simulink library "vmc"  (R2021b)
settings: Solver=VariableStepAuto  StartTime=0.0  StopTime=10.0  RelTol=1e-3
undefined symbols (not defined in the file or in its folder): AVMC_ACCDeltaTqIGain_X_kph, AVMC_ACCDeltaTqIGain_Y_mps2, AVMC_ACCDeltaTqIGainP2_X_kph, AVMC_ACCDeltaTqIGainP2_Y_mps2, AVMC_ACCDeltaTqPGain_X_kph, AVMC_ACCDeltaTqPGain_Y_kph, AVMC_ACCDeltaTqPGainP2_X_kph, AVMC_ACCDeltaTqPGainP2_Y_kph, AVMC_ACCLongSteadyCtrl_X_kph, AVMC_CCAccelCMD_X_kph, AVMC_CCAccelCMD_Y_kph, AVMC_CCDeltaTqIGain_X_kph, AVMC_CCDeltaTqIGain_Y_mps2, AVMC_CCDeltaTqPGain_X_kph, AVMC_CCDeltaTqPGain_Y_kph, AVMC_CCLongSteadyCtrl_X_kph, AVMC_DISCDeltaTqIGainP2_X_kph, AVMC_DISCDeltaTqIGainP2_Y_mps2, AVMC_ESCRegenOut_X_kph, AVMC_ESCRegenOut_Y_Deg, AVMC_ESCRegenOutEnSpd_X_Deg, AVMC_LatESCRegenOut_X_kph, AVMC_LatESCRegenOut_Y_Deg, AVMC_LongAccDeadZone_X_kph, AVMC_LongAccDeadZoneP2_X_kph, AVMC_LongAccFiltTs_X_Gps, AVMC_LongAccFiltTsP2_X_Gps, AVMC_MCPresBaseTq_X_bar, AVMC_MSAAccelCMD_X_kph, AVMC_MSAAccelCMD_Y_kph, AVMC_MSADeltaTqIGain_X_kph, AVMC_MSADeltaTqIGain_Y_mps2, AVMC_MSADeltaTqPGain_X_kph, AVMC_MSADeltaTqPGain_Y_kph, AVMC_MSALongSteadyCtrl_X_kph, AVMC_MSAPedalOvrd_X_kph, AVMC_MSASpdBand_X_kph, AVMC_OPDDisSlideRate_X_Deg, AVMC_RDCDetectTime_X_kph, AVMC_RDCDetectTime_Y_pct, AVMC_RDCEnSlideRate_X_Deg, AVMC_StESCYaw_X_kph, AVMC_StESCYaw_Y_Deg, AVMC_StESCYawCom_X_kph, AVMC_StESCYawCom_Y_Gps, AVMC_TMSpdBaseTq_X_rpm, C_TASK_10MS_S, C_TASK_5MS_S, DEG2RAD, Discrete, ENUM_ADASACCSTA_ACTIVE, ENUM_ADASACCSTA_OVERRIDE, ENUM_ADASACCSTA_STANDBY, ENUM_ADASMSASTA_ACTIVE, ENUM_ADASMSASTA_ERROR, ENUM_ADASMSASTA_OFF, ENUM_ADASMSASTA_OVERSPEED, ENUM_ADASMSASTA_STANDBY, ENUM_ADASMSASTA_UNDERSPEED, ENUM_ADASMSASTA_UNLIMIT ... (+254)
libraries: hcu_lib x57, simulink x49, ctrlSharedLib x6, simulink_extras x1
(part 5 of 9)

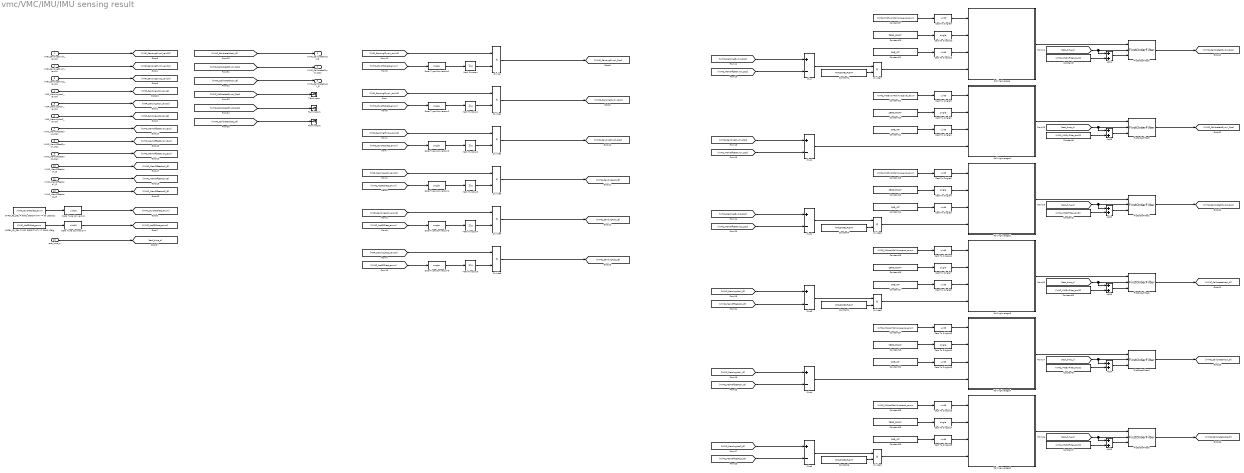
== system vmc/VMC/IMU/IMU sensing result  ==
  VINP_SensingGyroX_raw16 : Inport
  VINP_SensingGyroY_raw16 : Inport  Port=2
  VINP_SensingGyroZ_raw16 : Inport  Port=3
  VINP_SensingAccX_raw16 : Inport  Port=4
  VINP_SensingAccY_raw16 : Inport  Port=5
  VINP_SensingAccZ_raw16 : Inport  Port=6
  VVMC_MemOffsetGyroX_Dps : Inport  Port=7
  VVMC_MemOffsetGyroY_Dps : Inport  Port=8
  VVMC_MemOffsetGyroZ_Dps : Inport  Port=9
  VVMC_MemOffsetAccX_G : Inport  Port=10
  VVMC_MemOffsetAccY_G : Inport  Port=11
  VVMC_MemOffsetAccZ_G : Inport  Port=12
  task_time_s : Inport  Port=13
  ACCEL_FS_SEL = 001 SENSITIVITY = 2000 LSB/g : Constant  Value=KVMC_AccFSSlect_enum
  Add{1..5,8} (6 alike) : Sum
  Cast To Single{1,4,7,10,14,17} (6 alike) : DataTypeConversion  OutDataTypeStr=single
  Cast To Single{2..3,5..6,8..9,11..13,15..16,18} (12 alike) : DataTypeConversion  OutDataTypeStr=uint8
  Constant{1..2,4,6} (4 alike) : Constant  Value=MINUSONE_FLOAT
  Constant{10,13,16,19..20,25} (6 alike) : Constant  Value=ZERO_FLOAT
  Constant{11,14,17,21..22,26} (6 alike) : Constant  Value=ONE_INT
  Constant12 : Constant  Value=KVMC_IMUGyroYRollAveLevel_enum
  Constant15 : Constant  Value=KVMC_IMUGyroZRollAveLevel_enum
  Constant18 : Constant  Value=KVMC_IMUAccXRollAveLevel_enum
  Constant23 : Constant  Value=KVMC_IMUGxFilter_raw32
  Constant24 : Constant  Value=KVMC_IMUAccYRollAveLevel_enum
  Constant27 : Constant  Value=KVMC_IMUGyroXRollAveLevel_enum
  Constant28 : Constant  Value=KVMC_IMUAccZRollAveLevel_enum
  Constant3 : Constant  Value=KVMC_IMURxFilter_raw32
  Constant5 : Constant  Value=KVMC_IMURzFilter_raw32
  Constant7 : Constant  Value=KVMC_IMUGzFilter_raw32
  Constant8 : Constant  Value=KVMC_IMUGyFilter_raw32
  Constant9 : Constant  Value=KVMC_IMURyFilter_raw32
  Data Type Conversion : DataTypeConversion  OutDataTypeStr=uint16
  Data Type Conversion{1..6} (6 alike) : DataTypeConversion  OutDataTypeStr=single
  Data Type Conversion7 : DataTypeConversion  OutDataTypeStr=uint16
  Divide{,1..9} (10 alike) : Product  Inputs=**
  FirstOrderFilter{1..6} (6 alike) : hcu_lib/Basic_Blocks/FirstOrderFilter
  GYRO_FS_SEL = 0001 SENSITIVITY = 50 LSB/dps : Constant  Value=KVMC_GyroFSSlect_enum
  Math Function{,1..5} (6 alike) : Math  Operator=reciprocal  SaturateOnIntegerOverflow=on
  Plus{,1..5} (6 alike) : Sum  Inputs=+-
  RollingAverage : Stateflow chart  TreatAsAtomicUnit=on
  RollingAverage1 : Stateflow chart  TreatAsAtomicUnit=on
  RollingAverage2 : Stateflow chart  TreatAsAtomicUnit=on
  RollingAverage3 : Stateflow chart  TreatAsAtomicUnit=on
  RollingAverage4 : Stateflow chart  TreatAsAtomicUnit=on
  RollingAverage5 : Stateflow chart  TreatAsAtomicUnit=on
  Terminator : Terminator
  Terminator1 : Terminator
  Terminator2 : Terminator
  VVMC_CalibratedAccX_G : Outport
  VVMC_CalibratedGyroY_Dps : Outport  Port=2
  VVMC_CalibratedAccY_G : Outport  Port=3
  wires:
  Divide4/1 -> [VVMC_SensingAccY_G]  "VVMC_SensingAccY_G"
  Divide3/1 -> [VVMC_SensingAccX_G]  "VVMC_SensingAccX_G"
  Divide2/1 -> [VVMC_SensingGyroZ_Dps]  "VVMC_SensingGyroZ_Dps"
  Divide1/1 -> [VVMC_SensingGyroY_Dps]  "VVMC_SensingGyroY_Dps"
  ACCEL_FS_SEL = 001 SENSITIVITY = 2000 LSB/g/1 -> Data Type Conversion7/1
  Data Type Conversion7/1 -> [VVMC_AccFSSlect_enum]  "VVMC_AccFSSlect_enum"
  [VINP_SensingAccZ_raw16] -> Divide5/1
  [VVMC_AccFSSlect_enum] -> Data Type Conversion5/1
  [VINP_SensingAccY_raw16] -> Divide4/1
  [VINP_SensingAccX_raw16] -> Divide3/1
  [VVMC_GyroFSSlect_enum] -> Data Type Conversion3/1
  [VINP_SensingGyroZ_raw16] -> Divide2/1
  [VINP_SensingGyroY_raw16] -> Divide1/1
  [VVMC_GyroFSSlect_enum] -> Data Type Conversion2/1
  Data Type Conversion/1 -> [VVMC_GyroFSSlect_enum]  "VVMC_GyroFSSlect_enum"
  GYRO_FS_SEL = 0001 SENSITIVITY = 50 LSB/dps/1 -> Data Type Conversion/1
  [VVMC_GyroFSSlect_enum] -> Data Type Conversion1/1
  [VINP_SensingGyroX_raw16] -> Divide/1
  VVMC_MemOffsetGyroY_Dps/1 -> [VVMC_MemOffsetGyroY_Dps]
  VVMC_MemOffsetGyroX_Dps/1 -> [VVMC_MemOffsetGyroX_Dps]
  VVMC_MemOffsetAccY_G/1 -> [VVMC_MemOffsetAccY_G]
  VVMC_MemOffsetAccZ_G/1 -> [VVMC_MemOffsetAccZ_G]
  VVMC_MemOffsetGyroZ_Dps/1 -> [VVMC_MemOffsetGyroZ_Dps]
  VVMC_MemOffsetAccX_G/1 -> [VVMC_MemOffsetAccX_G]
  VINP_SensingGyroX_raw16/1 -> [VINP_SensingGyroX_raw16]
  VINP_SensingGyroY_raw16/1 -> [VINP_SensingGyroY_raw16]
  VINP_SensingGyroZ_raw16/1 -> [VINP_SensingGyroZ_raw16]
  VINP_SensingAccX_raw16/1 -> [VINP_SensingAccX_raw16]
  VINP_SensingAccY_raw16/1 -> [VINP_SensingAccY_raw16]
  VINP_SensingAccZ_raw16/1 -> [VINP_SensingAccZ_raw16]
  Divide5/1 -> [VVMC_SensingAccZ_G]  "VVMC_SensingAccZ_G"
  Divide/1 -> [VVMC_SensingGyroX_Dps]  "VVMC_SensingGyroX_Dps"
  [VVMC_SensingGyroX_Dps] -> Plus/1
  [VVMC_MemOffsetGyroX_Dps] -> Plus/2
  [VVMC_SensingGyroY_Dps] -> Plus1/1
  [VVMC_MemOffsetGyroY_Dps] -> Plus1/2
  [VVMC_SensingGyroZ_Dps] -> Plus2/1
  [VVMC_MemOffsetGyroZ_Dps] -> Plus2/2
  [VVMC_SensingAccX_G] -> Plus3/1
  [VVMC_MemOffsetAccX_G] -> Plus3/2
  [VVMC_SensingAccY_G] -> Plus4/1
  [VVMC_MemOffsetAccY_G] -> Plus4/2
  [VVMC_SensingAccZ_G] -> Plus5/1
  [VVMC_MemOffsetAccZ_G] -> Plus5/2
  FirstOrderFilter1/1 -> [VVMC_CalibratedGyroX_Dps]  "VVMC_CalibratedGyroX_Dps"
  FirstOrderFilter5/1 -> [VVMC_CalibratedGyroY_Dps]  "VVMC_CalibratedGyroY_Dps"
  FirstOrderFilter2/1 -> [VVMC_CalibratedGyroZ_Dps]  "VVMC_CalibratedGyroZ_Dps"
  FirstOrderFilter6/1 -> [VVMC_CalibratedAccX_G]  "VVMC_CalibratedAccX_G"
  FirstOrderFilter4/1 -> [VVMC_CalibratedAccY_G]  "VVMC_CalibratedAccY_G"
  FirstOrderFilter3/1 -> [VVMC_CalibratedAccZ_G]  "VVMC_CalibratedAccZ_G"
  Math Function/1 -> Divide/2
  Math Function1/1 -> Divide1/2
  Math Function2/1 -> Divide2/2
  Math Function3/1 -> Divide3/2
  Math Function4/1 -> Divide4/2
  Math Function5/1 -> Divide5/2
  Data Type Conversion1/1 -> Math Function/1
  Data Type Conversion2/1 -> Math Function1/1
  Data Type Conversion3/1 -> Math Function2/1
  [VVMC_AccFSSlect_enum] -> Data Type Conversion4/1
  Data Type Conversion4/1 -> Math Function3/1
  Data Type Conversion5/1 -> Math Function4/1
  [VVMC_AccFSSlect_enum] -> Data Type Conversion6/1
  Data Type Conversion6/1 -> Math Function5/1
  task_time_s/1 -> [task_time_s]
  [task_time_s] -> Add8/1, FirstOrderFilter6/2
  Plus3/1 -> Divide6/1
  Constant23/1 -> Add8/2
  Add8/1 -> FirstOrderFilter6/3
  Constant1/1 -> Divide6/2
  Divide6/1 -> RollingAverage3/4(VINP_INPData_raw32)
  Divide7/1 -> RollingAverage/4(VINP_INPData_raw32)
  Constant2/1 -> Divide7/2
  Add1/1 -> FirstOrderFilter1/3
  Constant3/1 -> Add1/2
  [task_time_s] -> FirstOrderFilter1/2, Add1/1
  Plus/1 -> Divide7/1
  [task_time_s] -> Add2/1, FirstOrderFilter2/2
  Constant5/1 -> Add2/2
  Add2/1 -> FirstOrderFilter2/3
  Constant4/1 -> Divide8/2
  Divide8/1 -> RollingAverage2/4(VINP_INPData_raw32)
  Plus2/1 -> Divide8/1
  Divide9/1 -> RollingAverage5/4(VINP_INPData_raw32)
  Constant6/1 -> Divide9/2
  Add3/1 -> FirstOrderFilter3/3
  Constant7/1 -> Add3/2
  [task_time_s] -> FirstOrderFilter3/2, Add3/1
  Plus5/1 -> Divide9/1
  Add4/1 -> FirstOrderFilter4/3
  Constant8/1 -> Add4/2
  [task_time_s] -> FirstOrderFilter4/2, Add4/1
  Plus4/1 -> RollingAverage4/4(VINP_INPData_raw32)
  [task_time_s] -> Add5/1, FirstOrderFilter5/2
  Constant9/1 -> Add5/2
  Add5/1 -> FirstOrderFilter5/3
  Plus1/1 -> RollingAverage1/4(VINP_INPData_raw32)
  Constant20/1 -> Cast To Single10/1
  Constant27/1 -> Cast To Single9/1
  Cast To Single12/1 -> RollingAverage/3(ONE_INT)
  Cast To Single9/1 -> RollingAverage/1(KVMC_RollAveLevel_enum)
  Cast To Single10/1 -> RollingAverage/2(ZERO_FLOAT)
  Constant21/1 -> Cast To Single12/1
  RollingAverage/1(VVMC_RollAve_raw32) -> FirstOrderFilter1/1
  Constant11/1 -> Cast To Single2/1
  Cast To Single1/1 -> RollingAverage1/2(ZERO_FLOAT)
  Cast To Single3/1 -> RollingAverage1/1(KVMC_RollAveLevel_enum)
  Cast To Single2/1 -> RollingAverage1/3(ONE_INT)
  Constant12/1 -> Cast To Single3/1
  Constant10/1 -> Cast To Single1/1
  RollingAverage1/1(VVMC_RollAve_raw32) -> FirstOrderFilter5/1
  Constant13/1 -> Cast To Single4/1
  Constant15/1 -> Cast To Single6/1
  Constant14/1 -> Cast To Single5/1
  Cast To Single6/1 -> RollingAverage2/1(KVMC_RollAveLevel_enum)
  Cast To Single4/1 -> RollingAverage2/2(ZERO_FLOAT)
  Cast To Single5/1 -> RollingAverage2/3(ONE_INT)
  RollingAverage2/1(VVMC_RollAve_raw32) -> FirstOrderFilter2/1
  Constant17/1 -> Cast To Single8/1
  Cast To Single7/1 -> RollingAverage3/2(ZERO_FLOAT)
  Cast To Single11/1 -> RollingAverage3/1(KVMC_RollAveLevel_enum)
  Cast To Single8/1 -> RollingAverage3/3(ONE_INT)
  Constant18/1 -> Cast To Single11/1
  Constant16/1 -> Cast To Single7/1
  RollingAverage3/1(VVMC_RollAve_raw32) -> FirstOrderFilter6/1
  Constant19/1 -> Cast To Single14/1
  Constant24/1 -> Cast To Single13/1
  Cast To Single15/1 -> RollingAverage4/3(ONE_INT)
  Cast To Single13/1 -> RollingAverage4/1(KVMC_RollAveLevel_enum)
  Cast To Single14/1 -> RollingAverage4/2(ZERO_FLOAT)
  Constant22/1 -> Cast To Single15/1
  RollingAverage4/1(VVMC_RollAve_raw32) -> FirstOrderFilter4/1
  Constant26/1 -> Cast To Single18/1
  Cast To Single17/1 -> RollingAverage5/2(ZERO_FLOAT)
  Cast To Single16/1 -> RollingAverage5/1(KVMC_RollAveLevel_enum)
  Cast To Single18/1 -> RollingAverage5/3(ONE_INT)
  Constant28/1 -> Cast To Single16/1
  Constant25/1 -> Cast To Single17/1
  RollingAverage5/1(VVMC_RollAve_raw32) -> FirstOrderFilter3/1
  [VVMC_CalibratedAccY_G] -> VVMC_CalibratedAccY_G/1
  [VVMC_CalibratedGyroY_Dps] -> VVMC_CalibratedGyroY_Dps/1
  [VVMC_CalibratedAccX_G] -> VVMC_CalibratedAccX_G/1
  [VVMC_CalibratedGyroX_Dps] -> Terminator/1
  [VVMC_CalibratedGyroZ_Dps] -> Terminator1/1
  [VVMC_CalibratedAccZ_G] -> Terminator2/1

== system vmc/VMC/Long Acceleration Calculation/Estimate Slope ==
  VINP_LongAccel_Gps : Inport
  VINP_VehSpeed_kph : Inport  Port=2
  task_time_s : Inport  Port=3
  VINP_GRADE_deg : Inport  Port=4
  VINP_DIDGetDynoMode_flg : Inport  Port=5
  VVMC_CalibratedAccX_G : Inport  Port=6
  AND5 : Logic  AllPortsSameDT=off  OutDataTypeStr=boolean
  Add : Sum  Inputs=+-
  Asin : Trigonometry  Operator=asin
  Constant1 : Constant  Value=KVMC_EstSlopeTs_c
  Constant14 : Constant  Value=KVMC_DIDGetDynoModeSW_flg
  Constant2 : Constant  Value=KVMC_EstSlopeTs_c
  Constant3 : Constant  Value=KVMC_EstSlopeTs_c
  Constant4 : Constant  Value=KVMC_EstSlopeSW_flg
  Constant5 : Constant  Value=KVMC_EstSlopeLongGSW_flg
  Constant6 : Constant  Value=ZERO_FLOAT
  FirstOrderFilter : hcu_lib/Basic_Blocks/FirstOrderFilter
  FirstOrderFilter1 : hcu_lib/Basic_Blocks/FirstOrderFilter
  FirstOrderFilter2 : hcu_lib/Basic_Blocks/FirstOrderFilter
  Gain : Gain  Gain=KPH2MPS
  Gain1 : Gain  Gain=1/GRAVITY_G
  Gain2 : Gain  Gain=RAD2DEG
  Switch : Switch  Criteria=u2 > Threshold
  Switch1 : Switch  Criteria=u2 > Threshold
  Switch2 : Switch  Criteria=u2 > Threshold
  derivative : hcu_lib/Basic_Blocks/derivative
  VVMC_EstSlope_Deg : Outport
  wires:
  VINP_VehSpeed_kph/1 -> FirstOrderFilter1/1
  Gain/1 -> derivative/1
  Gain1/1 -> Add/2
  Add/1 -> Asin/1  "sum"
  FirstOrderFilter/1 -> Add/1
  FirstOrderFilter1/1 -> Gain/1
  derivative/1 -> Gain1/1
  Asin/1 -> Gain2/1
  Gain2/1 -> FirstOrderFilter2/1
  FirstOrderFilter2/1 -> Switch/1  "VVMC_CalEstSlope_Deg"
  Switch1/1 -> VVMC_EstSlope_Deg/1  "VVMC_EstSlope_Deg"
  task_time_s/1 -> [task_time_s]
  [task_time_s] -> FirstOrderFilter/2
  Constant1/1 -> FirstOrderFilter/3
  [task_time_s] -> FirstOrderFilter2/2
  Constant3/1 -> FirstOrderFilter2/3
  Constant2/1 -> FirstOrderFilter1/3
  [task_time_s] -> FirstOrderFilter1/2
  Constant4/1 -> Switch/2
  VINP_GRADE_deg/1 -> Switch/3
  [task_time_s] -> derivative/2
  Constant14/1 -> AND5/2
  Switch/1 -> Switch1/3
  AND5/1 -> Switch1/2
  Constant6/1 -> Switch1/1
  VINP_DIDGetDynoMode_flg/1 -> [VINP_DIDGetDynoMode_flg]
  [VINP_DIDGetDynoMode_flg] -> AND5/1
  Switch2/1 -> FirstOrderFilter/1
  VINP_LongAccel_Gps/1 -> Switch2/3
  VVMC_CalibratedAccX_G/1 -> Switch2/1
  Constant5/1 -> Switch2/2

== system vmc/VMC/Long Acceleration Calculation/Vehicle to Meter Speed ==
  InputSpeed : Inport
  Add : Sum
  Constant1 : Constant  Value=KVMC_Veh2MetSpdAdd_kph
  Constant11 : Constant  Value=KVMC_Veh2MetSpdGain_c
  Product : Product
  OutputSpeed : Outport
  wires:
  InputSpeed/1 -> Product/1
  Product/1 -> Add/1
  Constant11/1 -> Product/2
  Add/1 -> OutputSpeed/1
  Constant1/1 -> Add/2

== system vmc/VMC/Long Acceleration Calculation/Wheel speed to long accelerate calculation ==
  VVMC_LFWhlSpeedRollAve_kph : Inport
  VVMC_RFWhlSpeedRollAve_kph : Inport  Port=2
  VVMC_LRWhlSpeedRollAve_kph : Inport  Port=3
  VVMC_RRWhlSpeedRollAve_kph : Inport  Port=4
  Add2 : Sum
  Add3 : Sum  Inputs=+-
  Constant10 : Constant  Value=KPH2MPS
  Constant11 : Constant  Value=KVMC_WSSCMDCycleTime_s
  Constant14 : Constant  Value=KVMC_GravityValue_mps2
  Constant9 : Constant  Value=KVMC_WhlSpdAvgNum_c
  Divide : Product  Inputs=*/
  Divide1 : Product  Inputs=**
  Divide2 : Product  Inputs=*/
  Divide3 : Product  Inputs=*/
  Terminator : Terminator
  Terminator1 : Terminator
  Unit Delay : UnitDelay  SampleTime=-1  HasFrameUpgradeWarning=on
  VVMC_WhlSpd2LongAcc_Gps : Outport
  wires:
  Constant11/1 -> Divide2/2
  Divide1/1 -> Divide2/1
  [VVMC_LFWhlSpeedRollAve_kph] -> Add2/1
  Constant9/1 -> Divide/2
  Divide/1 -> Add3/1, Unit Delay/1
  Divide2/1 -> Divide3/1
  [VVMC_RFWhlSpeedRollAve_kph] -> Add2/2
  Constant10/1 -> Divide1/2
  Add3/1 -> Divide1/1
  Unit Delay/1 -> Add3/2
  Add2/1 -> Divide/1
  Constant14/1 -> Divide3/2
  Divide3/1 -> VVMC_WhlSpd2LongAcc_Gps/1  "VVMC_WhlSpd2LongAcc_Gps"
  VVMC_LFWhlSpeedRollAve_kph/1 -> [VVMC_LFWhlSpeedRollAve_kph]
  VVMC_RFWhlSpeedRollAve_kph/1 -> [VVMC_RFWhlSpeedRollAve_kph]
  VVMC_LRWhlSpeedRollAve_kph/1 -> Terminator/1
  VVMC_RRWhlSpeedRollAve_kph/1 -> Terminator1/1

== system vmc/VMC/Long Acceleration Calculation/WheelSpeedRollingAverage ==
  VINP_LFRawWhlSpeed_kph : Inport
  VINP_RFRawWhlSpeed_kph : Inport  Port=2
  VINP_LRRawWhlSpeed_kph : Inport  Port=3
  VINP_RRRawWhlSpeed_kph : Inport  Port=4
  Constant : Constant  Value=ONE_INT
  Constant1 : Constant  Value=KVMC_WhlSpdRollAveLevel_enum
  Constant2 : Constant  Value=ZERO_FLOAT
  WheelSpeedRollingAverage : Stateflow chart  TreatAsAtomicUnit=on
  VVMC_LFWhlSpeedRollAve_kph : Outport
  VVMC_RFWhlSpeedRollAve_kph : Outport  Port=2
  VVMC_LRWhlSpeedRollAve_kph : Outport  Port=3
  VVMC_RRWhlSpeedRollAve_kph : Outport  Port=4
  wires:
  [VINP_LFRawWhlSpeed_kph] -> WheelSpeedRollingAverage/1(VINP_LFRawWhlSpeed_kph)
  [VINP_RRRawWhlSpeed_kph] -> WheelSpeedRollingAverage/4(VINP_RRRawWhlSpeed_kph)
  [VINP_RFRawWhlSpeed_kph] -> WheelSpeedRollingAverage/2(VINP_RFRawWhlSpeed_kph)
  WheelSpeedRollingAverage/4(VVMC_RRWhlSpeedRollAve_kph) -> [VVMC_RRWhlSpeedRollAve_kph]
  WheelSpeedRollingAverage/2(VVMC_RFWhlSpeedRollAve_kph) -> [VVMC_RFWhlSpeedRollAve_kph]
  Constant/1 -> WheelSpeedRollingAverage/5(ONE_INT)
  Constant1/1 -> WheelSpeedRollingAverage/6(KVMC_WhlSpdRollAveLevel_enum)
  [VINP_LRRawWhlSpeed_kph] -> WheelSpeedRollingAverage/3(VINP_LRRawWhlSpeed_kph)
  WheelSpeedRollingAverage/1(VVMC_LFWhlSpeedRollAve_kph) -> [VVMC_LFWhlSpeedRollAve_kph]
  Constant2/1 -> WheelSpeedRollingAverage/7(ZERO_FLOAT)
  WheelSpeedRollingAverage/3(VVMC_LRWhlSpeedRollAve_kph) -> [VVMC_LRWhlSpeedRollAve_kph]
  VINP_LRRawWhlSpeed_kph/1 -> [VINP_LRRawWhlSpeed_kph]
  VINP_RRRawWhlSpeed_kph/1 -> [VINP_RRRawWhlSpeed_kph]
  VINP_LFRawWhlSpeed_kph/1 -> [VINP_LFRawWhlSpeed_kph]
  VINP_RFRawWhlSpeed_kph/1 -> [VINP_RFRawWhlSpeed_kph]
  [VVMC_LFWhlSpeedRollAve_kph] -> VVMC_LFWhlSpeedRollAve_kph/1
  [VVMC_RFWhlSpeedRollAve_kph] -> VVMC_RFWhlSpeedRollAve_kph/1
  [VVMC_LRWhlSpeedRollAve_kph] -> VVMC_LRWhlSpeedRollAve_kph/1
  [VVMC_RRWhlSpeedRollAve_kph] -> VVMC_RRWhlSpeedRollAve_kph/1

== system vmc/VMC/LongAccel_EstSlope/Estimate Slope ==
  VINP_LongAccel_Gps : Inport
  VINP_VehSpeed_kph : Inport  Port=2
  VINP_GRADE_deg : Inport  Port=3
  Add : Sum  Inputs=+-
  Asin : Trigonometry  Operator=asin
  Constant1 : Constant  Value=KVMC_EstSlopeLongAccelTs_c
  Constant2 : Constant  Value=KVMC_EstSlopeVehSpdTs_c
  Constant3 : Constant  Value=KVMC_EstSlopeTs_c
  Constant4 : Constant  Value=KVMC_EstSlopeSW_flg
  Constant{5..8} (4 alike) : Constant  Value=C_TASK_10MS_S
  FirstOrderFilter : hcu_lib/Basic_Blocks/FirstOrderFilter
  FirstOrderFilter1 : hcu_lib/Basic_Blocks/FirstOrderFilter
  FirstOrderFilter2 : hcu_lib/Basic_Blocks/FirstOrderFilter
  Gain : Gain  Gain=KPH2MPS
  Gain1 : Gain  Gain=1/GRAVITY_G
  Gain2 : Gain  Gain=RAD2DEG
  Switch : Switch  Criteria=u2 > Threshold
  derivative : hcu_lib/Basic_Blocks/derivative
  VVMC_EstSlope_Deg : Outport
  wires:
  VINP_VehSpeed_kph/1 -> FirstOrderFilter1/1
  Gain/1 -> derivative/1
  VINP_LongAccel_Gps/1 -> FirstOrderFilter/1
  Gain1/1 -> Add/2
  Add/1 -> Asin/1  "sum"
  FirstOrderFilter/1 -> Add/1
  FirstOrderFilter1/1 -> Gain/1
  derivative/1 -> Gain1/1
  Asin/1 -> Gain2/1
  Gain2/1 -> FirstOrderFilter2/1
  FirstOrderFilter2/1 -> Switch/1
  Switch/1 -> VVMC_EstSlope_Deg/1
  Constant5/1 -> FirstOrderFilter/2
  Constant1/1 -> FirstOrderFilter/3
  Constant7/1 -> FirstOrderFilter2/2
  Constant3/1 -> FirstOrderFilter2/3
  Constant2/1 -> FirstOrderFilter1/3
  Constant6/1 -> FirstOrderFilter1/2
  Constant4/1 -> Switch/2
  VINP_GRADE_deg/1 -> Switch/3
  Constant8/1 -> derivative/2

== system vmc/VMC/LongAccel_EstSlope/VehSpdRollingAverage ==
  VINP_VehSpeed_kph : Inport
  Constant3 : Constant  Value=ONE_INT
  Constant4 : Constant  Value=KVMC_VehSpdRollAveLevel_enum
  Constant5 : Constant  Value=ZERO_FLOAT
  RollingAverage : Stateflow chart  TreatAsAtomicUnit=on
  VVMC_VehSpdRollAve_kph : Outport
  wires:
  [VVMC_VehSpdRollAve_kph] -> VVMC_VehSpdRollAve_kph/1
  VINP_VehSpeed_kph/1 -> [VINP_VehSpeed_kph]  "VINP_VehSpeed_kph"
  RollingAverage/1(VVMC_VehSpdRollAve_kph) -> [VVMC_VehSpdRollAve_kph]  "VVMC_VehSpdRollAve_kph"
  [VINP_VehSpeed_kph] -> RollingAverage/4(VINP_VehSpeed_kph)
  Constant3/1 -> RollingAverage/3(ONE_INT)
  Constant5/1 -> RollingAverage/2(ZERO_FLOAT)
  Constant4/1 -> RollingAverage/1(KVMC_VehSpdRollAveLevel_enum)

== system vmc/VMC/MSA function/Anti-Speed Limitation ==
  VINP_HoodSW_flg : Inport
  VTQD_GearActualPosn_enum : Inport  Port=2
  VINP_ZoneSpdCrlMode_enum : Inport  Port=3
  VINP_SetSpd_kph : Inport  Port=4
  AND : Logic  Inputs=3  AllPortsSameDT=off  OutDataTypeStr=boolean
  Constant1 : Constant  Value=KVMC_AntiSpdLimSW_flg
  Constant2 : Constant  Value=ENUM_GEARACTUALPOSN_D
  Constant4 : Constant  Value=3  OutDataTypeStr=uint8
  Constant5 : Constant  Value=KVMC_AntiSpdLim_kph
  Equal : RelationalOperator  Operator===  OutDataTypeStr=boolean  RndMeth=Simplest
  Switch : Switch  Criteria=u2 > Threshold
  Switch1 : Switch  Criteria=u2 > Threshold
  VVMC_AntiSpdLimEn_flg : Outport
  VVMC_MSASpdCtrlMode_enum : Outport  Port=2
  VVMC_MSASetSpd_kph : Outport  Port=3
  wires:
  [VINP_HoodSW_flg] -> AND/1
  Constant1/1 -> AND/3
  Equal/1 -> AND/2
  AND/1 -> [VVMC_AntiSpdLimEn_flg]  "VVMC_AntiSpdLimEn_flg"
  [VVMC_AntiSpdLimEn_flg] -> Switch/2
  [VINP_ZoneSpdCrlMode_enum] -> Switch/3
  [VINP_SetSpd_kph] -> Switch1/3
  Constant4/1 -> Switch/1
  [VVMC_AntiSpdLimEn_flg] -> Switch1/2
  Switch1/1 -> [VVMC_MSASetSpd_kph]  "VVMC_MSASetSpd_kph"
  Switch/1 -> [VVMC_MSASpdCtrlMode_enum]  "VVMC_MSASpdCtrlMode_enum"
  Constant2/1 -> Equal/2
  Constant5/1 -> Switch1/1
  [VTQD_GearActualPosn_enum] -> Equal/1
  VINP_HoodSW_flg/1 -> [VINP_HoodSW_flg]
  [VVMC_AntiSpdLimEn_flg] -> VVMC_AntiSpdLimEn_flg/1
  [VVMC_MSASpdCtrlMode_enum] -> VVMC_MSASpdCtrlMode_enum/1
  [VVMC_MSASetSpd_kph] -> VVMC_MSASetSpd_kph/1
  VTQD_GearActualPosn_enum/1 -> [VTQD_GearActualPosn_enum]
  VINP_ZoneSpdCrlMode_enum/1 -> [VINP_ZoneSpdCrlMode_enum]
  VINP_SetSpd_kph/1 -> [VINP_SetSpd_kph]

== system vmc/VMC/MSA function/MSAActivationHandshake ==
  VVMC_MSASpdCtrlMode_enum : Inport
  VTQD_ExternalTqAllow_flg : Inport  Port=2
  VINP_VehSpeed_kph : Inport  Port=3
  VVMC_MSASetSpd_kph : Inport  Port=4
  VINP_SWCCANCELSta_flg : Inport  Port=5
  VVMC_MSAUnLimit_flg : Inport  Port=6
  VTQD_GearActualPosn_enum : Inport  Port=7
  VINP_SWCResUpSta_flg : Inport  Port=8
  VINP_SWCSetdownSta_flg : Inport  Port=9
  VVMC_AntiSpdLimEn_flg : Inport  Port=10
  VVMC_CalMeterSpeed_kph : Inport  Port=11
  Chart : Stateflow chart  TreatAsAtomicUnit=on
  Constant : Constant  Value=KVMC_MSAActiveMetSpdHi_kph
  Constant1 : Constant  Value=KVMC_MSAActiveMetSpdLo_kph
  Constant2 : Constant  Value=KVMC_CCMSASpdWar_kph
  Constant3 : Constant  Value=ZERO_INT
  Data Type Conversion : DataTypeConversion  OutDataTypeStr=uint8
  Delay : Delay  DelayLength=1
  Detect Decrease{1..4} (4 alike) : simulink/Logic and Bit Operations/Detect Decrease  vinit=0.0  OutDataTypeStr=boolean
  Logical Operator : Logic  Operator=OR  AllPortsSameDT=off  OutDataTypeStr=boolean
  MVMC_MSASpdBand_Y_kph : Lookup_n-D  NumberOfTableDimensions=1  BreakpointsForDimension1=AVMC_MSASpdBand_X_kph  Table=MVMC_MSASpdBand_Y_kph  ExtrapMethod=Clip  InternalRulePriority=Speed  RndMeth=Simplest  InputSameDT=on
  Saturation Dynamic : simulink/Discontinuities/Saturation Dynamic  OutMin=[]  OutMax=[]  OutDataTypeStr=Inherit: Same as second input  OutDataType=fixdt(1, 16)  OutScaling=2^-10  DoSatur=off
  Switch : Switch  Criteria=u2 > Threshold
  VVMC_MSACtrlSta_enum : Outport
  VVMC_MSASpdWar_flg : Outport  Port=2
  VVMC_MSAActive_flg : Outport  Port=3
  wires:
  Chart/1(VVMC_MSACtrlSta_enum) -> [VVMC_MSACtrlSta_enum]  "VVMC_MSACtrlSta_enum"
  Chart/3(VVMC_MSAActive_flg) -> [VVMC_MSAActive_flg]  "VVMC_MSAActive_flg"
  Chart/2(VVMC_MSASpdWar_flg) -> [VVMC_MSASpdWar_flg]  "VVMC_MSASpdWar_flg"
  [VVMC_MSASpdBand_kph] -> Chart/9(VVMC_MSASpdBand_kph)
  VINP_VehSpeed_kph/1 -> [VINP_VehSpeed_kph]
  VINP_SWCCANCELSta_flg/1 -> [VINP_SWCCANCELSta_flg]
  VTQD_ExternalTqAllow_flg/1 -> [VTQD_ExternalTqAllow_flg]
  VVMC_MSASpdCtrlMode_enum/1 -> [VVMC_MSASpdCtrlMode_enum]
  [VVMC_MSAActive_flg] -> VVMC_MSAActive_flg/1
  [VVMC_MSASpdWar_flg] -> VVMC_MSASpdWar_flg/1
  [VVMC_MSACtrlSta_enum] -> VVMC_MSACtrlSta_enum/1
  [VINP_SWCCANCELSta_flg] -> Detect Decrease1/1
  Constant2/1 -> Chart/7(KVMC_CCMSASpdWar_kph)
  [VVMC_MSASetSpd_kph] -> Data Type Conversion/1
  [VINP_VehSpeed_kph] -> Chart/4(VINP_VehSpeed_kph)
  Constant/1 -> Chart/3(KVMC_MSAActiveMetSpdHi_kph)
  [VTQD_ExternalTqAllow_flg] -> Chart/2(VTQD_ExternalTqAllow_flg)
  [VVMC_MSASpdCtrlMode_enum] -> Chart/1(VVMC_MSASpdCtrlMode_enum)
  [VVMC_MSAUnLimit_flg] -> Delay/1
  Delay/1 -> Chart/10(VVMC_MSAUnLimit_flg)
  VVMC_MSAUnLimit_flg/1 -> [VVMC_MSAUnLimit_flg]
  VTQD_GearActualPosn_enum/1 -> [VTQD_GearActualPosn_enum]
  [VTQD_GearActualPosn_enum] -> Chart/11(VTQD_GearActualPosn_enum)
  Saturation Dynamic/1 -> [VVMC_MSASpdBand_kph]  "VVMC_MSASpdBand_kph"
  MVMC_MSASpdBand_Y_kph/1 -> Saturation Dynamic/2
  Constant3/1 -> Saturation Dynamic/3
  VINP_SWCSetdownSta_flg/1 -> [VINP_SWCSetdownSta_flg]
  VINP_SWCResUpSta_flg/1 -> [VINP_SWCResUpSta_flg]
  Detect Decrease2/1 -> Chart/12(VINP_SWCResUpSta_flg)
  Detect Decrease3/1 -> Chart/13(VINP_SWCSetdownSta_flg)
  [VINP_SWCResUpSta_flg] -> Detect Decrease2/1
  [VINP_SWCSetdownSta_flg] -> Detect Decrease3/1
  VVMC_AntiSpdLimEn_flg/1 -> [VVMC_AntiSpdLimEn_flg]
  Switch/1 -> Chart/5(VVMC_MSAActiveMetSpdLo_kph)
  [VVMC_MSASetSpd_kph] -> Switch/1
  [VVMC_AntiSpdLimEn_flg] -> Switch/2
  Constant1/1 -> Switch/3
  Data Type Conversion/1 -> Chart/6(VVMC_MSASetSpd_kph)
  [VVMC_MSASetSpd_kph] -> MVMC_MSASpdBand_Y_kph/1
  [VVMC_MSASetSpd_kph] -> Saturation Dynamic/1
  VVMC_MSASetSpd_kph/1 -> [VVMC_MSASetSpd_kph]
  [VVMC_AntiSpdLimEn_flg] -> Chart/14(VVMC_AntiSpdLimEn_flg)
  Logical Operator/1 -> Chart/8(VVMC_DetectSWCCANCEL_flg)  "VVMC_DetectSWCCANCEL_flg"
  [VVMC_AntiSpdLimEn_flg] -> Detect Decrease4/1
  Detect Decrease1/1 -> Logical Operator/1
  Detect Decrease4/1 -> Logical Operator/2
  VVMC_CalMeterSpeed_kph/1 -> [VVMC_CalMeterSpeed_kph]
  [VVMC_CalMeterSpeed_kph] -> Chart/15(VVMC_CalMeterSpeed_kph)

== system vmc/VMC/MSA function/MSADemandTorqueCalculation ==
  VVMC_MSASetSpd_kph : Inport
  VVMC_MSAActive_flg : Inport  Port=2
  VTQD_DriverWhlTqDem_Nm : Inport  Port=3
  VVMC_LongAcc_Gps : Inport  Port=4
  VVMC_MSAUnLimit_flg : Inport  Port=5
  VVMC_CalMeterSpeed_kph : Inport  Port=6
  " MSA Acceleration Determination" : Lookup_n-D  BreakpointsForDimension1=AVMC_MSAAccelCMD_Y_kph  BreakpointsForDimension2=AVMC_MSAAccelCMD_X_kph  BreakpointsForDimension3=[5, 7]  Table=MVMC_MSAAccelCMD_Z_mps2  ExtrapMethod=Clip  InternalRulePriority=Speed  RndMeth=Simplest  InputSameDT=on
      settings: InputPortMap=u0,u1
  Abs : Abs
  Add : Sum  Inputs=+-
  Add{1..2,5..6} (4 alike) : Sum
  Add3 : Sum  Inputs=+-
  Add4 : Sum  Inputs=+-
  Constant : Constant  Value=KVMC_MSAInitTqDEM_Nm
  Constant1 : Constant  Value=KVMC_MSAAccelCMDUpLim_mps2
  Constant10 : Constant  Value=KVMC_GravityValue_mps2
  Constant11 : Constant  Value=KVMC_MSADevLowLim_mps2
  Constant12 : Constant  Value=ZERO_INT
  Constant13 : Constant  Value=KVMC_MSAPGainTqSW_flg
  Constant14 : Constant  Value=KVMC_MSAPGainTqSW_flg
  Constant15 : Constant  Value=ZERO_INT
  Constant16 : Constant  Value=ZERO_INT
  Constant19 : Constant  Value=KVMC_MSADevUpLim_mps2
  Constant2 : Constant  Value=KVMC_MSAAccelCMDLowLim_mps2
  Constant3 : Constant  Value=KVMC_MSATqUpLim_Nm  OutDataTypeStr=single
  Constant4 : Constant  Value=KVMC_MSATqLowLim_Nm  OutDataTypeStr=single
  Constant5 : Constant  Value=KVMC_MSAPedalOvrdSetSpd_kph
  Constant6 : Constant  Value=KVMC_MSAIGainOffDevSpd_kph
  Constant7 : Constant  Value=KVMC_MSASpdDevUpLim_kph
  Constant8 : Constant  Value=KVMC_MSASpdDevLowLim_kph
  Detect Increase : simulink/Logic and Bit Operations/Detect Increase  vinit=0.0  OutDataTypeStr=boolean
  MVMC_MSADeltaTqIGain_Z_Nm : Lookup_n-D  BreakpointsForDimension1=AVMC_MSADeltaTqIGain_Y_mps2  BreakpointsForDimension2=AVMC_MSADeltaTqIGain_X_kph  Table=MVMC_MSADeltaTqIGain_Z_Nm  ExtrapMethod=Clip  InternalRulePriority=Speed  RndMeth=Simplest  InputSameDT=on
      settings: InputPortMap=u0,u1
  MVMC_MSADeltaTqPGain_Z_Nm : Lookup_n-D  BreakpointsForDimension1=AVMC_MSADeltaTqPGain_Y_kph  BreakpointsForDimension2=AVMC_MSADeltaTqPGain_X_kph  BreakpointsForDimension3=[5, 7]  Table=MVMC_MSADeltaTqPGain_Z_Nm  ExtrapMethod=Clip  InternalRulePriority=Speed  RndMeth=Simplest  InputSameDT=on
      settings: InputPortMap=u0,u1
  Product : Product
  Relational Operator : RelationalOperator  Operator=<  OutDataTypeStr=boolean  RndMeth=Simplest
  Saturation Dynamic{,1..2,4} (4 alike) : simulink/Discontinuities/Saturation Dynamic  OutMin=[]  OutMax=[]  OutDataTypeStr=Inherit: Same as second input  OutDataType=fixdt(1, 16)  OutScaling=2^-10  DoSatur=off
  Switch : Switch  Criteria=u2 ~= 0
  Switch1 : Switch  Criteria=u2 ~= 0
  Switch{2..5,7} (5 alike) : Switch  Criteria=u2 > Threshold
  Unit Delay : UnitDelay  SampleTime=-1  HasFrameUpgradeWarning=on
  VVMC_MSAWhlTqCal_Nm : Outport
  wires:
  Switch3/1 -> Add5/1  "VVMC_MSADeltaTqIGain_Nm"
  Add5/1 -> [VVMC_MSADeltaTq_Nm]  "VVMC_MSADeltaTq_Nm"
  Saturation Dynamic4/1 -> [VVMC_MSAActSpdDev_kph], MVMC_MSADeltaTqPGain_Z_Nm/1  "VVMC_MSAActSpdDev_kph"
  Constant8/1 -> Saturation Dynamic4/3
  Constant7/1 -> Saturation Dynamic4/1
  Add4/1 -> Saturation Dynamic4/2
  Add6/1 -> [VVMC_MSAWhlTqCal_Nm]  "VVMC_MSAWhlTqCal_Nm"
  Constant4/1 -> Saturation Dynamic/3
  Switch1/1 -> Saturation Dynamic/2
  Saturation Dynamic2/1 -> [VVMC_MSAAccelCMD_mps2]  "VVMC_MSAAccelCMD_mps2"
  " MSA Acceleration Determination"/1 -> Saturation Dynamic2/2
  Constant1/1 -> Saturation Dynamic2/1
  Constant2/1 -> Saturation Dynamic2/3
  Add3/1 -> Saturation Dynamic1/2
  [VVMC_LongAcc_Gps] -> Product/1
  Constant10/1 -> Product/2
  Constant19/1 -> Saturation Dynamic1/1
  Saturation Dynamic1/1 -> MVMC_MSADeltaTqIGain_Z_Nm/1  "VVMC_ActMSAAccDev_mps2"
  Product/1 -> Add3/2
  Constant11/1 -> Saturation Dynamic1/3
  [VVMC_MSAAccelCMD_mps2] -> Add3/1
  VVMC_LongAcc_Gps/1 -> [VVMC_LongAcc_Gps]
  VTQD_DriverWhlTqDem_Nm/1 -> [VTQD_DriverWhlTqDem_Nm]
  VVMC_MSAActive_flg/1 -> [VVMC_MSAActive_flg]
  VVMC_MSASetSpd_kph/1 -> [VVMC_MSASetSpd_kph]
  [VVMC_MSAWhlTqCal_Nm] -> VVMC_MSAWhlTqCal_Nm/1
  [VVMC_MSADeltaTq_Nm] -> Add2/2
  [VVMC_MSADeltaTq_Nm] -> Add1/2
  Switch/1 -> Switch1/1
  Add2/1 -> Switch/3
  Unit Delay/1 -> [VVMC_MSAWhlTqCalDelay_Nm]  "VVMC_MSAWhlTqCalDelay_Nm"
  Detect Increase/1 -> Switch/2
  [VVMC_MSAActive_flg] -> Switch1/2
  [VVMC_MSAActive_flg] -> Detect Increase/1
  Add1/1 -> Switch/1
  [VVMC_MSAWhlTqCalDelay_Nm] -> Add2/1
  [VTQD_DriverWhlTqDem_Nm] -> Add1/1
  Constant/1 -> Switch1/3
  Add/1 -> " MSA Acceleration Determination"/1
  VVMC_MSAUnLimit_flg/1 -> [VVMC_MSAUnLimit_flg]
  [VVMC_MSAUnLimit_flg] -> Switch2/2
  Constant5/1 -> Switch2/1
  Switch2/1 -> [VVMC_ActMSASetSpd_kph]  "VVMC_ActMSASetSpd_kph"
  [VVMC_ActMSASetSpd_kph] -> Add/1
  [VVMC_ActMSASetSpd_kph] -> Add4/1
  [VVMC_CalMeterSpeed_kph] -> Add/2
  [VVMC_CalMeterSpeed_kph] -> Add4/2
  VVMC_CalMeterSpeed_kph/1 -> [VVMC_CalMeterSpeed_kph]
  [VVMC_ActMSASetSpd_kph] -> " MSA Acceleration Determination"/2
  [VVMC_ActMSASetSpd_kph] -> MVMC_MSADeltaTqIGain_Z_Nm/2
  [VVMC_ActMSASetSpd_kph] -> MVMC_MSADeltaTqPGain_Z_Nm/2
  Constant3/1 -> Switch7/3
  [VVMC_MSAActive_flg] -> Switch7/2
  Switch7/1 -> Saturation Dynamic/1  "VVMC_MSATqUpLim_Nm"
  [VTQD_DriverWhlTqDem_Nm] -> Switch7/1
  [VVMC_MSASetSpd_kph] -> Switch2/3
  Switch4/1 -> Add6/1
  Constant14/1 -> Switch4/2
  [VVMC_MSADeltaTqPGain_Nm] -> Switch4/1
  Constant15/1 -> Switch4/3
  Saturation Dynamic/1 -> Unit Delay/1, Add6/2
  MVMC_MSADeltaTqPGain_Z_Nm/1 -> [VVMC_MSADeltaTqPGain_Nm]  "VVMC_MSADeltaTqPGain_Nm"
  [VVMC_MSADeltaTqPGain_Nm] -> Switch5/3
  Switch5/1 -> Add5/2
  Constant13/1 -> Switch5/2
  Constant16/1 -> Switch5/1
  Relational Operator/1 -> Switch3/2
  Abs/1 -> Relational Operator/1
  Constant6/1 -> Relational Operator/2
  [VVMC_MSAActSpdDev_kph] -> Abs/1
  Constant12/1 -> Switch3/1
  MVMC_MSADeltaTqIGain_Z_Nm/1 -> Switch3/3

== system vmc/VMC/MSA function/MSATorqueSourceDetermination ==
  VVMC_MSAWhlTqCal_Nm : Inport
  VTQD_DriverWhlTqDem_Nm : Inport  Port=2
  VVMC_MSACtrlSta_enum : Inport  Port=3
  VVMC_MSAActive_flg : Inport  Port=4
  VINP_VehSpeed_kph : Inport  Port=5
  VVMC_MSASetSpd_kph : Inport  Port=6
  task_time_s : Inport  Port=7
  VDHP_ActAPSPosn_pct : Inport  Port=8
  VVMC_AntiSpdLimEn_flg : Inport  Port=9
  AND : Logic  Inputs=3  AllPortsSameDT=off  OutDataTypeStr=boolean
  AND{2..6} (5 alike) : Logic  AllPortsSameDT=off  OutDataTypeStr=boolean
  Add1 : Sum  Inputs=+-
  Constant1 : Constant  Value=KVMC_MSAUnLimitDetTime_s
  Constant10 : Constant  Value=KVMC_MSAUnLimitResetTime_s
  Constant14 : Constant  Value=KVMC_MSAPedOvrdTqConTq_Nm
  Constant15 : Constant  Value=ENUM_ADASMSASTA_ACTIVE
  Constant3 : Constant  Value=ENUM_ADASMSASTA_ACTIVE
  Delay3 : Delay  DelayLength=1
  Detect Decrease : simulink/Logic and Bit Operations/Detect Decrease  vinit=0.0  OutDataTypeStr=boolean
  Detect Increase1 : simulink/Logic and Bit Operations/Detect Increase  vinit=0.0  OutDataTypeStr=boolean
  Equal1 : RelationalOperator  Operator===  OutDataTypeStr=boolean  RndMeth=Simplest
  Equal2 : RelationalOperator  Operator===  OutDataTypeStr=boolean  RndMeth=Simplest
  MVMC_MSAPedalOvrd_Y_pct : Lookup_n-D  NumberOfTableDimensions=1  BreakpointsForDimension1=AVMC_MSAPedalOvrd_X_kph  Table=MVMC_MSAPedalOvrd_Y_pct  ExtrapMethod=Clip  InternalRulePriority=Speed  RndMeth=Simplest  InputSameDT=on
  NOT{,2..5} (5 alike) : Logic  Operator=NOT  AllPortsSameDT=off  OutDataTypeStr=boolean
  OR : Logic  Operator=OR  Inputs=3  AllPortsSameDT=off  OutDataTypeStr=boolean
  OR3 : Logic  Operator=OR  AllPortsSameDT=off  OutDataTypeStr=boolean
  Relational Operator : RelationalOperator  OutDataTypeStr=boolean  RndMeth=Simplest
  Relational Operator1 : RelationalOperator  Operator=>  OutDataTypeStr=boolean  RndMeth=Simplest
  Relational Operator2 : RelationalOperator  OutDataTypeStr=boolean  RndMeth=Simplest
  Relational Operator3 : RelationalOperator  Operator=<=  OutDataTypeStr=boolean  RndMeth=Simplest
  Relational Operator4 : RelationalOperator  OutDataTypeStr=boolean  RndMeth=Simplest
  Relational Operator5 : RelationalOperator  Operator=<=  OutDataTypeStr=boolean  RndMeth=Simplest
  SR_Latch1 : hcu_lib/Basic_Blocks/SR_Latch
  SR_Latch2 : hcu_lib/Basic_Blocks/SR_Latch
  Switch : Switch  Criteria=u2 ~= 0
  Timer : hcu_lib/Basic_Blocks/Timer
  Timer1 : hcu_lib/Basic_Blocks/Timer
  VVMC_MSAWhlTqReq_Nm : Outport
  VVMC_MSAUnLimit_flg : Outport  Port=2
  wires:
  [VVMC_MSAWhlTqCal_Nm] -> Relational Operator/1
  [VTQD_DriverWhlTqDem_Nm] -> Relational Operator/2
  [VTQD_DriverWhlTqDem_Nm] -> Switch/1
  [VVMC_MSAWhlTqCal_Nm] -> Switch/3
  Switch/1 -> [VVMC_MSAWhlTqReq_Nm]  "VVMC_MSAWhlTqReq_Nm"
  [VVMC_MSAWhlTqReq_Nm] -> VVMC_MSAWhlTqReq_Nm/1
  VVMC_MSAWhlTqCal_Nm/1 -> [VVMC_MSAWhlTqCal_Nm]
  VTQD_DriverWhlTqDem_Nm/1 -> [VTQD_DriverWhlTqDem_Nm]
  Constant1/1 -> Relational Operator2/2, Timer/4
  VVMC_MSACtrlSta_enum/1 -> [VVMC_MSACtrlSta_enum]
  Timer/1 -> Relational Operator2/1  "VVMC_MSAUnLimitDetTime_s"
  Relational Operator2/1 -> [VVMC_MSAUnLimitDetFinish_flg]  "VVMC_MSAUnLimitDetFinish_flg"
  NOT/1 -> Timer/2
  [task_time_s] -> Timer/3
  SR_Latch1/1 -> [VVMC_MSAUnLimit_flg]  "VVMC_MSAUnLimit_flg"
  [VINP_VehSpeed_kph] -> Relational Operator3/1
  NOT2/1 -> OR/1
  [VVMC_MSAActive_flg] -> NOT2/1
  OR/1 -> SR_Latch1/2  "VVMC_MASUnLimitDis_flg"
  OR3/1 -> Switch/2  "VVMC_MSAChangeToPedal_flg"
  [VVMC_ActMSAUnLimit_flg] -> OR3/2
  VVMC_MSAActive_flg/1 -> [VVMC_MSAActive_flg]
  VINP_VehSpeed_kph/1 -> [VINP_VehSpeed_kph]
  VVMC_MSASetSpd_kph/1 -> [VVMC_MSASetSpd_kph]
  task_time_s/1 -> [task_time_s]
  [VVMC_MSAUnLimit_flg] -> VVMC_MSAUnLimit_flg/1
  AND2/1 -> OR/2
  Relational Operator3/1 -> AND2/1
  [VVMC_MSAUnLimit_flg] -> Delay3/1
  Delay3/1 -> Timer1/1, NOT3/1
  NOT3/1 -> Timer1/2
  [task_time_s] -> Timer1/3
  Constant10/1 -> Relational Operator4/2, Timer1/4
  Timer1/1 -> Relational Operator4/1  "VVMC_MSAUnLimitResetTime_s"
  Relational Operator4/1 -> [VVMC_MSAUnLimitReset_flg]  "VVMC_MSAUnLimitReset_flg"
  [VVMC_MSAUnLimitReset_flg] -> AND2/2
  VDHP_ActAPSPosn_pct/1 -> [VDHP_ActAPSPosn_pct]
  MVMC_MSAPedalOvrd_Y_pct/1 -> Relational Operator1/2  "VVMC_MSAPedalOvrd_pct"
  [VDHP_ActAPSPosn_pct] -> Relational Operator1/1
  [VVMC_MSAUnLimitDetFinish_flg] -> SR_Latch1/1
  [VTQD_DriverWhlTqDem_Nm] -> Add1/1
  [VVMC_MSAWhlTqCal_Nm] -> Add1/2
  [VVMC_MSAUnLimit_flg] -> AND3/2
  Relational Operator5/1 -> AND3/1
  Constant14/1 -> Relational Operator5/2
  Add1/1 -> Relational Operator5/1
  Relational Operator/1 -> AND4/2
  NOT4/1 -> AND4/1
  [VVMC_MSAUnLimit_flg] -> NOT4/1
  AND4/1 -> OR3/1
  Relational Operator1/1 -> AND5/1, Detect Increase1/1, Detect Decrease/1
  SR_Latch2/1 -> AND5/2  "VVMC_MSAInstPedOvrd_flg"
  Detect Decrease/1 -> SR_Latch2/2
  Constant15/1 -> Equal1/2
  [VVMC_MSACtrlSta_enum] -> Equal1/1
  AND6/1 -> SR_Latch2/1
  Detect Increase1/1 -> AND6/1
  Equal1/1 -> AND6/2
  AND5/1 -> [VVMC_MSAPedalOvrd_flg]  "VVMC_MSAPedalOvrd_flg"
  [VVMC_MSASetSpd_kph] -> MVMC_MSAPedalOvrd_Y_pct/1
  [VVMC_MSASetSpd_kph] -> Relational Operator3/2
  VVMC_AntiSpdLimEn_flg/1 -> [VVMC_AntiSpdLimEn_flg]
  AND3/1 -> [VVMC_ActMSAUnLimit_flg]  "VVMC_ActMSAUnLimit_flg"
  [VVMC_AntiSpdLimEn_flg] -> NOT5/1
  Constant3/1 -> Equal2/2
  [VVMC_MSAPedalOvrd_flg] -> AND/1
  AND/1 -> NOT/1, Timer/1  "VVMC_UnLimitTimerEn_flg"
  Equal2/1 -> AND/3
  NOT5/1 -> AND/2
  [VVMC_MSACtrlSta_enum] -> Equal2/1
  [VVMC_AntiSpdLimEn_flg] -> OR/3

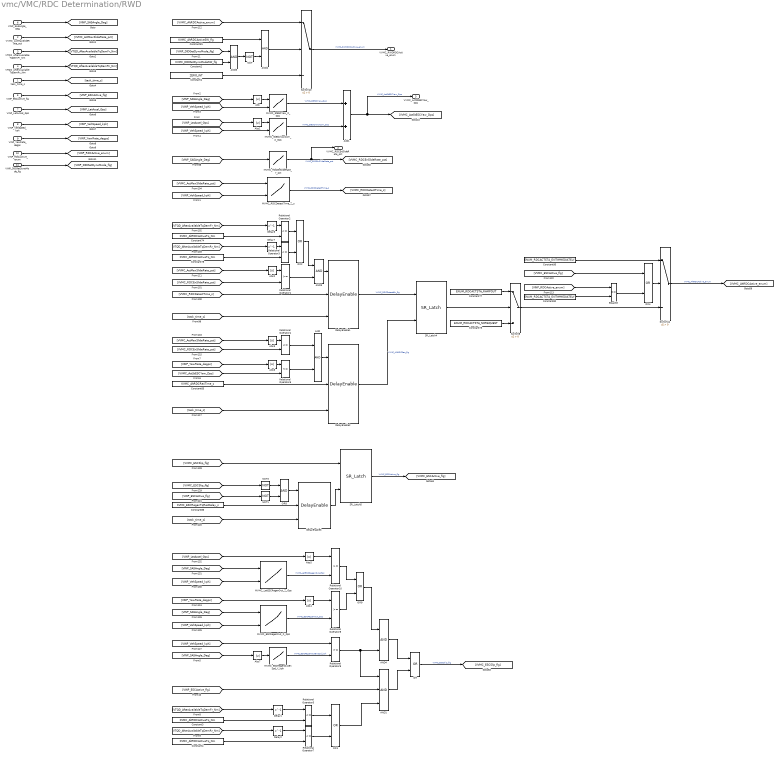
== system vmc/VMC/RDC Determination/RWD ==
  task_time_s : Inport
  VVMC_ActMaxSlideRate_pct : Inport  Port=2
  VTQD_AfterAvailableTqDemFr_Nm : Inport  Port=3
  VTQD_AfterAvailableTqDemRr_Nm : Inport  Port=4
  VINP_ESCActive_flg : Inport  Port=5
  VINP_SASAngle_Deg : Inport  Port=6
  VINP_LatAccel_Gps : Inport  Port=7
  VINP_VehSpeed_kph : Inport  Port=8
  VINP_YawRate_degps : Inport  Port=9
  VINP_RDCActive_enum : Inport  Port=10
  VINP_DIDGetDynoMode_flg : Inport  Port=11
  AND{,2..5} (5 alike) : Logic  AllPortsSameDT=off  OutDataTypeStr=boolean
  AND1 : Logic  Inputs=3  AllPortsSameDT=off  OutDataTypeStr=boolean
  Abs{,1..7} (8 alike) : Abs
  Add1 : Sum
  Constant1 : Constant  Value=ZERO_INT
  Constant2 : Constant  Value=KVMC_DIDGetDynoModeSW_flg
  Constant{3..4,74,78} (4 alike) : Constant  Value=KVMC_AltRDCActiveTq_Nm
  Constant73 : Constant  Value=ENUM_RDCACTSTA_NOREQUEST
  Constant77 : Constant  Value=ENUM_RDCACTSTA_RAMPOUT
  Constant81 : Constant  Value=KVMC_AltRDCActiveSW_flg
  Constant82 : Constant  Value=ENUM_RDCACTSTA_EXITIMMEDIATELY
  Constant83 : Constant  Value=KVMC_AltRDCRecTime_s
  Constant86 : Constant  Value=KVMC_ESCRegenTqRecDelay_s
  Constant95 : Constant  Value=ENUM_RDCACTSTA_EXITIMMEDIATELY
  Delay{1..2,6..7} (4 alike) : Delay  DelayLength=1
  DelayEnable1 : hcu_lib/Basic_Blocks/DelayEnable
  DelayEnable2 : hcu_lib/Basic_Blocks/DelayEnable
  DelayEnable3 : hcu_lib/Basic_Blocks/DelayEnable
  Equal33 : RelationalOperator  Operator===  OutDataTypeStr=boolean  RndMeth=Simplest
  MVMC_ESCRegenOutEnSpd_Y_kph : Lookup_n-D  NumberOfTableDimensions=1  BreakpointsForDimension1=AVMC_ESCRegenOutEnSpd_X_Deg  Table=MVMC_ESCRegenOutEnSpd_Y_kph  ExtrapMethod=Clip  InternalRulePriority=Speed  RndMeth=Simplest  InputSameDT=on
  MVMC_ESCRegenOut_Z_Dps : Lookup_n-D  BreakpointsForDimension1=AVMC_ESCRegenOut_Y_Deg  BreakpointsForDimension2=AVMC_ESCRegenOut_X_kph  Table=MVMC_ESCRegenOut_Z_Dps  ExtrapMethod=Clip  InternalRulePriority=Speed  RndMeth=Simplest  InputSameDT=on
      settings: InputPortMap=u0,u1
  MVMC_LatESCRegenOut_Z_Gps : Lookup_n-D  BreakpointsForDimension1=AVMC_LatESCRegenOut_Y_Deg  BreakpointsForDimension2=AVMC_LatESCRegenOut_X_kph  Table=MVMC_LatESCRegenOut_Z_Gps  ExtrapMethod=Clip  InternalRulePriority=Speed  RndMeth=Simplest  InputSameDT=on
      settings: InputPortMap=u0,u1
  MVMC_RDCDetectTime_Z_s : Lookup_n-D  BreakpointsForDimension1=AVMC_RDCDetectTime_Y_pct  BreakpointsForDimension2=AVMC_RDCDetectTime_X_kph  Table=MVMC_RDCDetectTime_Z_s  ExtrapMethod=Clip  InternalRulePriority=Speed  RndMeth=Simplest  InputSameDT=on
      settings: InputPortMap=u0,u1
  MVMC_RDCEnSlideRate_Y_pct : Lookup_n-D  NumberOfTableDimensions=1  BreakpointsForDimension1=AVMC_RDCEnSlideRate_X_Deg  Table=MVMC_RDCEnSlideRate_Y_pct  ExtrapMethod=Clip  InternalRulePriority=Speed  RndMeth=Simplest  InputSameDT=on
  MVMC_StESCYawCom_Z_Dps : Lookup_n-D  BreakpointsForDimension1=AVMC_StESCYawCom_Y_Gps  BreakpointsForDimension2=AVMC_StESCYawCom_X_kph  Table=MVMC_StESCYawCom_Z_Dps  ExtrapMethod=Clip  InternalRulePriority=Speed  RndMeth=Simplest  InputSameDT=on
      settings: InputPortMap=u0,u1
  MVMC_StESCYaw_Z_Dps : Lookup_n-D  BreakpointsForDimension1=AVMC_StESCYaw_Y_Deg  BreakpointsForDimension2=AVMC_StESCYaw_X_kph  Table=MVMC_StESCYaw_Z_Dps  ExtrapMethod=Clip  InternalRulePriority=Speed  RndMeth=Simplest  InputSameDT=on
      settings: InputPortMap=u0,u1
  NOT : Logic  Operator=NOT  AllPortsSameDT=off  OutDataTypeStr=boolean
  NOT1 : Logic  Operator=NOT  AllPortsSameDT=off  OutDataTypeStr=boolean
  NOT3 : Logic  Operator=NOT  AllPortsSameDT=off  OutDataTypeStr=boolean
  OR{,1..2,4,9} (5 alike) : Logic  Operator=OR  AllPortsSameDT=off  OutDataTypeStr=boolean
  OR8 : Logic  AllPortsSameDT=off  OutDataTypeStr=boolean
  Relational Operator{1,8..10} (4 alike) : RelationalOperator  OutDataTypeStr=boolean  RndMeth=Simplest
  Relational Operator{2..7} (6 alike) : RelationalOperator  Operator=<=  OutDataTypeStr=boolean  RndMeth=Simplest
  SR_Latch4 : hcu_lib/Basic_Blocks/SR_Latch
  SR_Latch5 : hcu_lib/Basic_Blocks/SR_Latch
  Switch10 : Switch  Criteria=u2 > Threshold
  Switch11 : Switch  Criteria=u2 > Threshold
  Switch8 : Switch  Criteria=u2 > Threshold
  VVMC_RWDRDCActive_enum : Outport
  VVMC_RDCEnSlideRate_pct : Outport  Port=2
  VVMC_ActStESCYaw_Dps : Outport  Port=3
  wires:
  [VVMC_RDCDetectTime_s] -> DelayEnable1/2
  MVMC_RDCEnSlideRate_Y_pct/1 -> VVMC_RDCEnSlideRate_pct/1, [VVMC_RDCEnSlideRate_pct]  "VVMC_RDCEnSlideRate_pct"
  VINP_YawRate_degps/1 -> [VINP_YawRate_degps]
  [VINP_ESCActive_flg] -> NOT1/1
  VINP_ESCActive_flg/1 -> [VINP_ESCActive_flg]
  OR2/1 -> AND3/1
  Constant73/1 -> Switch8/3
  Delay7/1 -> Relational Operator3/1
  VINP_LatAccel_Gps/1 -> [VINP_LatAccel_Gps]
  [VVMC_RDCEnSlideRate_pct] -> Relational Operator1/2
  Switch11/1 -> [VVMC_AltRDCActive_enum]  "VVMC_AltRDCActive_enum"
  VINP_VehSpeed_kph/1 -> [VINP_VehSpeed_kph]
  Constant78/1 -> Relational Operator3/2
  [VINP_SASAngle_Deg] -> Abs7/1
  VVMC_ActMaxSlideRate_pct/1 -> [VVMC_ActMaxSlideRate_pct]
  DelayEnable2/1 -> SR_Latch4/2  "VVMC_AltRDCRec_flg"
  [task_time_s] -> DelayEnable1/3
  OR9/1 -> AND4/1
  [VINP_SASAngle_Deg] -> MVMC_LatESCRegenOut_Z_Gps/1
  [VVMC_ActMaxSlideRate_pct] -> MVMC_RDCDetectTime_Z_s/1
  [VINP_LatAccel_Gps] -> Abs5/1
  VTQD_AfterAvailableTqDemRr_Nm/1 -> [VTQD_AfterAvailableTqDemRr_Nm]
  SR_Latch5/1 -> [VVMC_ESCActive_flg]  "VVMC_ESCActive_flg"
  Abs4/1 -> Relational Operator8/1
  DelayEnable1/1 -> SR_Latch4/1  "VVMC_RDCDetectEn_flg"
  Relational Operator8/1 -> OR9/2
  Constant74/1 -> Relational Operator2/2
  [VVMC_ESCSlip_flg] -> SR_Latch5/1
  Abs5/1 -> Relational Operator10/1
  [VINP_SASAngle_Deg] -> MVMC_ESCRegenOut_Z_Dps/1
  [VINP_VehSpeed_kph] -> Relational Operator9/1
  Switch8/1 -> Switch11/3
  NOT3/1 -> OR8/1
  [VTQD_AfterAvailableTqDemFr_Nm] -> Delay6/1
  Delay6/1 -> Relational Operator2/1
  MVMC_RDCDetectTime_Z_s/1 -> [VVMC_RDCDetectTime_s]  "VVMC_RDCDetectTime_s"
  [VTQD_AfterAvailableTqDemRr_Nm] -> Delay7/1
  [VINP_SASAngle_Deg] -> MVMC_RDCEnSlideRate_Y_pct/1
  AND3/1 -> DelayEnable1/1
  [VVMC_ESCActive_flg] -> OR4/1
  Relational Operator3/1 -> OR2/2
  Relational Operator9/1 -> AND4/2, AND1/1
  Relational Operator1/1 -> AND3/2
  MVMC_ESCRegenOut_Z_Dps/1 -> Relational Operator8/2  "VVMC_ESCRegenOut_Dps"
  [VINP_YawRate_degps] -> Abs4/1
  SR_Latch4/1 -> Switch8/2
  [VVMC_ActMaxSlideRate_pct] -> Abs2/1
  Switch10/1 -> VVMC_RWDRDCActive_enum/1  "VVMC_RWDRDCActive_enum"
  [VINP_RDCActive_enum] -> Equal33/1
  VINP_SASAngle_Deg/1 -> [VINP_SASAngle_Deg]
  [task_time_s] -> DelayEnable3/3
  Abs2/1 -> Relational Operator1/1
  MVMC_LatESCRegenOut_Z_Gps/1 -> Relational Operator10/2  "VVMC_LatESCRegenOut_Gps"
  NOT1/1 -> OR8/2
  Equal33/1 -> OR4/2
  [VINP_VehSpeed_kph] -> MVMC_LatESCRegenOut_Z_Gps/2
  [VVMC_ESCSlip_flg] -> NOT3/1
  Relational Operator2/1 -> OR2/1
  Relational Operator10/1 -> OR9/1
  Constant95/1 -> Switch11/1
  [VINP_VehSpeed_kph] -> MVMC_ESCRegenOut_Z_Dps/2
  OR8/1 -> DelayEnable3/1
  OR4/1 -> Switch11/2
  [VVMC_AltRDCActive_enum] -> Switch10/1
  DelayEnable3/1 -> SR_Latch5/2
  Constant77/1 -> Switch8/1
  Constant86/1 -> DelayEnable3/2
  Constant82/1 -> Equal33/2
  VTQD_AfterAvailableTqDemFr_Nm/1 -> [VTQD_AfterAvailableTqDemFr_Nm]
  VINP_RDCActive_enum/1 -> [VINP_RDCActive_enum]
  task_time_s/1 -> [task_time_s]
  Constant1/1 -> Switch10/3
  [VINP_LatAccel_Gps] -> Abs1/1
  [VINP_SASAngle_Deg] -> Abs/1
  Abs/1 -> MVMC_StESCYaw_Z_Dps/1
  Add1/1 -> VVMC_ActStESCYaw_Dps/1, [VVMC_ActStESCYaw_Dps]  "VVMC_ActStESCYaw_Dps"
  MVMC_StESCYaw_Z_Dps/1 -> Add1/1  "VVMC_StESCYaw_Dps"
  [VINP_VehSpeed_kph] -> MVMC_StESCYaw_Z_Dps/2
  [VINP_VehSpeed_kph] -> MVMC_StESCYawCom_Z_Dps/2
  MVMC_StESCYawCom_Z_Dps/1 -> Add1/2  "VVMC_StESCYawCom_Dps"
  Abs1/1 -> MVMC_StESCYawCom_Z_Dps/1
  [VINP_VehSpeed_kph] -> MVMC_RDCDetectTime_Z_s/2
  AND/1 -> DelayEnable2/1
  [task_time_s] -> DelayEnable2/3
  Relational Operator4/1 -> AND/1
  [VVMC_ActStESCYaw_Dps] -> Relational Operator6/2
  [VVMC_RDCEnSlideRate_pct] -> Relational Operator4/2
  Abs6/1 -> Relational Operator6/1
  Relational Operator6/1 -> AND/2
  Abs3/1 -> Relational Operator4/1
  [VVMC_ActMaxSlideRate_pct] -> Abs3/1
  Constant83/1 -> DelayEnable2/2
  [VINP_YawRate_degps] -> Abs6/1
  Abs7/1 -> MVMC_ESCRegenOutEnSpd_Y_kph/1
  MVMC_ESCRegenOutEnSpd_Y_kph/1 -> Relational Operator9/2  "VVMC_ESCRegenOutEnSpd_kph"
  Constant4/1 -> Relational Operator7/2
  Delay1/1 -> Relational Operator5/1
  [VTQD_AfterAvailableTqDemRr_Nm] -> Delay2/1
  Constant3/1 -> Relational Operator5/2
  Delay2/1 -> Relational Operator7/1
  Relational Operator7/1 -> OR1/2
  Relational Operator5/1 -> OR1/1
  [VTQD_AfterAvailableTqDemFr_Nm] -> Delay1/1
  OR1/1 -> AND1/3
  [VINP_ESCActive_flg] -> AND1/2
  AND4/1 -> OR/1
  AND1/1 -> OR/2
  OR/1 -> [VVMC_ESCSlip_flg]  "VVMC_ESCSlip_flg"
  Constant81/1 -> AND2/1
  AND2/1 -> Switch10/2
  VINP_DIDGetDynoMode_flg/1 -> [VINP_DIDGetDynoMode_flg]
  [VINP_DIDGetDynoMode_flg] -> AND5/1
  Constant2/1 -> AND5/2
  AND5/1 -> NOT/1
  NOT/1 -> AND2/2
